simulink model "gm_parallel_8_phase_voltages"  (R2022a)
settings: Solver=FixedStepDiscrete  StartTime=0.0  StopTime=10.0  RelTol=1e-3
undefined symbols (not defined in the file or in its folder): f_c, u_dc
libraries: hdlmdlgenlib x14, simulink x2
(part 1 of 4)
settings Model: Creator=Andre Merx  LastModifiedBy=Andre Merx
settings SolverCC: AlgebraicLoopSolver=TrustRegion
settings DataIOCC: LimitDataPoints=on  SaveOutput=off  SaveTime=off
settings OptimizationCC: BlockReduction=off  ConditionallyExecuteInputs=off  DefaultParameterBehavior=Inlined  LifeSpan=inf
settings DebuggingCC: AlgebraicLoopMsg=error  InheritedTsInSrcMsg=none  SingleTaskRateTransMsg=error  UnconnectedInputMsg=warning  UnconnectedOutputMsg=warning  UnconnectedLineMsg=warning  AllowSymbolicDim=off  StrictBusMsg=ErrorOnBusTreatedAsVector  SFUnexpectedBacktrackingDiag=warning  SFNoUnconditionalDefaultTransitionDiag=warning  SFExecutionAtInitializationDiag=none  SFMachineParentedDataDiag=warning  ArithmeticOperatorsInVariantConditions=warning
settings HardwareCC: ProdBitPerPointer=32  ProdBitPerSizeT=32  ProdBitPerPtrDiffT=32  ProdLargestAtomicFloat=None  ProdIntDivRoundTo=Undefined  ProdEndianess=Unspecified  ProdWordSize=32  ProdHWDeviceType=ASIC/FPGA->ASIC/FPGA  ProdEqTarget=off
settings SFSimCC: SimUseLocalCustomCode=off  CustomCodeUndefinedFunction=UseInterfaceOnly
settings RTWCC: RTWUseLocalCustomCode=off
settings CodeAppCC: StateflowObjectComments=on
settings GRTTargetCC: TargetLangStandard=C89/C90 (ANSI)
settings ConfigComp: CovScope=ReferencedModels  CovMetricSettings=dw  CovSaveCumulativeToWorkspaceVar=on  CovSaveSingleToWorkspaceVar=on  CovExternalEMLEnable=off  CovSFcnEnable=off

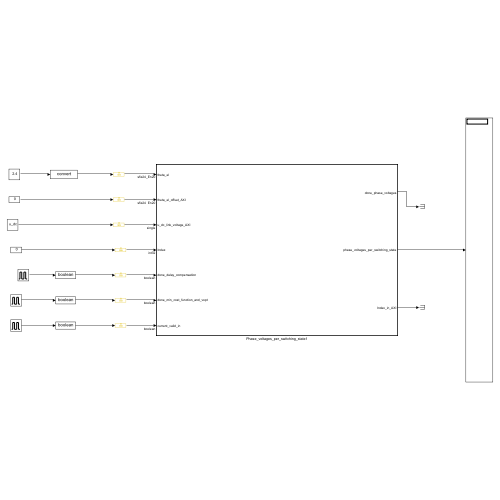
[thumbnail: Simulink's stored preview of the top-level diagram]
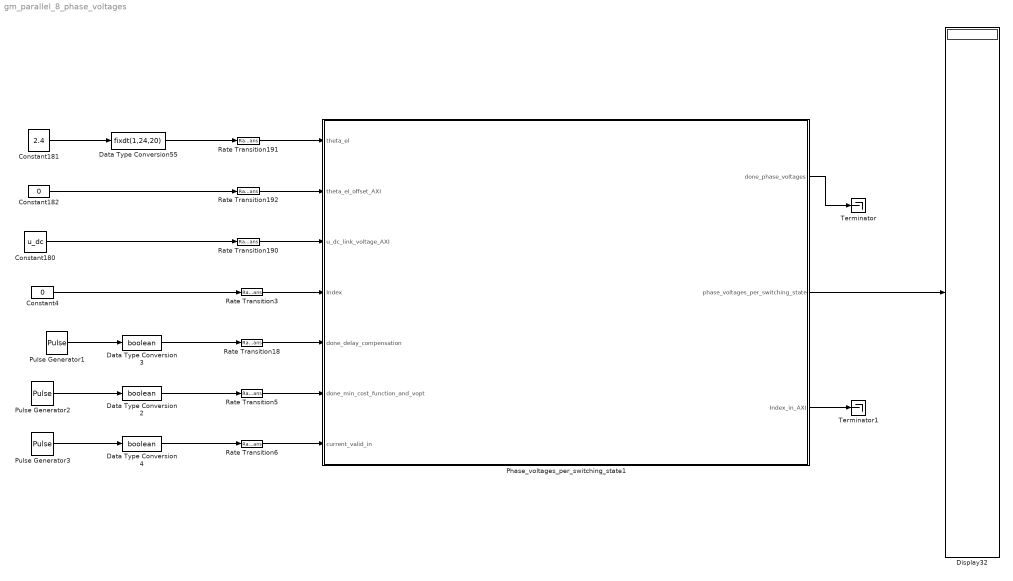
== system gm_parallel_8_phase_voltages ==
  Constant180 : Constant  Value=u_dc  OutDataTypeStr=single  SampleTime=-1
  Constant181 : Constant  Value=2.4
  Constant182 : Constant  Value=0  OutDataTypeStr=fixdt(1,24,20)  SampleTime=-1
  Constant4 : Constant  Value=0  OutDataTypeStr=int32  SampleTime=-1
  Data Type Conversion2 : DataTypeConversion  OutDataTypeStr=boolean  SaturateOnIntegerOverflow=off  RndMeth=Floor
  Data Type Conversion3 : DataTypeConversion  OutDataTypeStr=boolean  SaturateOnIntegerOverflow=off  RndMeth=Floor
  Data Type Conversion4 : DataTypeConversion  OutDataTypeStr=boolean  SaturateOnIntegerOverflow=off  RndMeth=Floor
  Data Type Conversion55 : DataTypeConversion  OutDataTypeStr=fixdt(1,24,20)  SaturateOnIntegerOverflow=off  RndMeth=Floor
  Display32 : Display
  Phase_voltages_per_switching_state1 : Subsystem  TreatAsAtomicUnit=on
  Pulse Generator1 : DiscretePulseGenerator  PulseType=Time based  Period=1/f_c
  Pulse Generator2 : DiscretePulseGenerator  PulseType=Time based  Period=1/f_c
  Pulse Generator3 : DiscretePulseGenerator  PulseType=Time based  Period=1/f_c
  Rate Transition{3,5..6,18,190..192} (7 alike) : RateTransition  OutPortSampleTime=Rt
  Terminator : Terminator
  Terminator1 : Terminator
  wires:
  Phase_voltages_per_switching_state1/3(Index_in_AXI) -> Terminator1/1
  Rate Transition3/1 -> Phase_voltages_per_switching_state1/4(Index)
  Data Type Conversion2/1 -> Rate Transition5/1
  Rate Transition6/1 -> Phase_voltages_per_switching_state1/7(current_valid_in)
  Rate Transition18/1 -> Phase_voltages_per_switching_state1/5(done_delay_compensation)
  Data Type Conversion3/1 -> Rate Transition18/1
  Data Type Conversion4/1 -> Rate Transition6/1
  Constant4/1 -> Rate Transition3/1
  Pulse Generator3/1 -> Data Type Conversion4/1
  Pulse Generator1/1 -> Data Type Conversion3/1
  Rate Transition5/1 -> Phase_voltages_per_switching_state1/6(done_min_cost_function_and_vopt)
  Pulse Generator2/1 -> Data Type Conversion2/1
  Phase_voltages_per_switching_state1/1(done_phase_voltages) -> Terminator/1
  Rate Transition190/1 -> Phase_voltages_per_switching_state1/3(u_dc_link_voltage_AXI)
  Rate Transition191/1 -> Phase_voltages_per_switching_state1/1(theta_el)
  Phase_voltages_per_switching_state1/2(phase_voltages_per_switching_state) -> Display32/1
  Rate Transition192/1 -> Phase_voltages_per_switching_state1/2(theta_el_offset_AXI)
  Constant182/1 -> Rate Transition192/1
  Constant180/1 -> Rate Transition190/1
  Data Type Conversion55/1 -> Rate Transition191/1
  Constant181/1 -> Data Type Conversion55/1

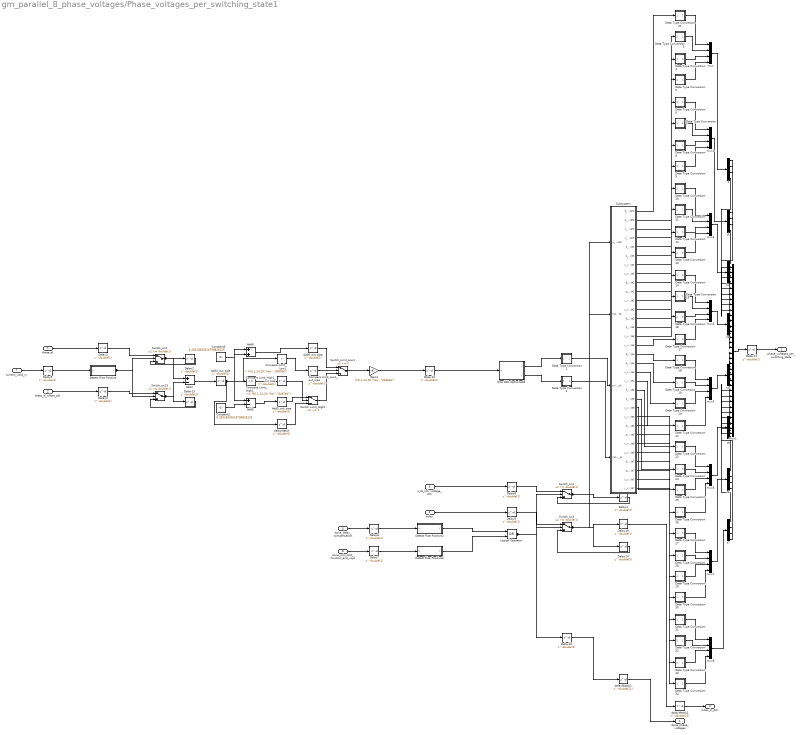
== system gm_parallel_8_phase_voltages/Phase_voltages_per_switching_state1 ==
  theta_el : Inport  OutDataTypeStr=fixdt(1, 24, 20)  PortDimensions=1  SampleTime=1e-08
  theta_el_offset_AXI : Inport  Port=2  OutDataTypeStr=fixdt(1, 24, 20)  PortDimensions=1  SampleTime=1e-08
  u_dc_link_voltage_AXI : Inport  Port=3  OutDataTypeStr=single  PortDimensions=1  SampleTime=1e-08
  Index : Inport  Port=4  OutDataTypeStr=int32  PortDimensions=1  SampleTime=1e-08
  done_delay_compensation : Inport  Port=5  OutDataTypeStr=boolean  PortDimensions=1  SampleTime=1e-08
  done_min_cost_function_and_vopt : Inport  Port=6  OutDataTypeStr=boolean  PortDimensions=1  SampleTime=1e-08
  current_valid_in : Inport  Port=7  OutDataTypeStr=boolean  PortDimensions=1  SampleTime=1e-08
  Add4 : Sum  Inputs=+-  AccumDataTypeStr=fixdt(1, 24, 20)  OutDataTypeStr=fixdt(1, 24, 20)  SampleTime=1e-08
  Add4_out_pipe : Delay  DelayLength=double(1)  InitialCondition=0  SampleTime=1e-08
  Add5 : Sum  Inputs=+-  AccumDataTypeStr=fixdt(1, 24, 20)  OutDataTypeStr=fixdt(1, 24, 20)  SampleTime=1e-08
  Add5_out_pipe : Delay  DelayLength=double(1)  InitialCondition=0  SampleTime=1e-08
  Add6 : Sum  AccumDataTypeStr=fixdt(1, 24, 20)  OutDataTypeStr=fixdt(1, 24, 20)  SampleTime=1e-08
  Add6_out_pipe : Delay  DelayLength=double(1)  InitialCondition=0  SampleTime=1e-08
  Compare Limit_High1 : simulink/Logic and Bit Operations/Compare To Constant  relop=>=  const="fi(0,1,24,20,\"hex\",\"6487ed\")"  OutDataTypeStr=boolean
  Compare Limit_High1_out_pipe : Delay  DelayLength=double(1)  InitialCondition=0  SampleTime=1e-08
  Compare Limit_Low1 : simulink/Logic and Bit Operations/Compare To Constant  relop=<  const="fi(0,1,24,20,\"hex\",\"000000\")"  OutDataTypeStr=boolean
  Compare Limit_Low1_out_pipe : Delay  DelayLength=double(1)  InitialCondition=0  SampleTime=1e-08
  Constant2 : Constant  Value=6.28318500518798828125  OutDataTypeStr=fixdt(1, 24, 20)  SampleTime=1e-08
  Constant3 : Constant  Value=6.28318500518798828125  OutDataTypeStr=fixdt(1, 24, 20)  SampleTime=1e-08
  Data Type Conversion1 : Subsystem
      mask Display: disp('NFP\nconv');
  Data Type Conversion10 : Subsystem
      mask Display: disp('NFP\nconv');
  Data Type Conversion11 : Subsystem
      mask Display: disp('NFP\nconv');
  Data Type Conversion12 : Subsystem
      mask Display: disp('NFP\nconv');
  Data Type Conversion13 : Subsystem
      mask Display: disp('NFP\nconv');
  Data Type Conversion14 : Subsystem
      mask Display: disp('NFP\nconv');
  Data Type Conversion15 : Subsystem
      mask Display: disp('NFP\nconv');
  Data Type Conversion16 : Subsystem
      mask Display: disp('NFP\nconv');
  Data Type Conversion17 : Subsystem
      mask Display: disp('NFP\nconv');
  Data Type Conversion18 : Subsystem
      mask Display: disp('NFP\nconv');
  Data Type Conversion19 : Subsystem
      mask Display: disp('NFP\nconv');
  Data Type Conversion2 : Subsystem
      mask Display: disp('NFP\nconv');
  Data Type Conversion20 : Subsystem
      mask Display: disp('NFP\nconv');
  Data Type Conversion21 : Subsystem
      mask Display: disp('NFP\nconv');
  Data Type Conversion22 : Subsystem
      mask Display: disp('NFP\nconv');
  Data Type Conversion23 : Subsystem
      mask Display: disp('NFP\nconv');
  Data Type Conversion24 : Subsystem
      mask Display: disp('NFP\nconv');
  Data Type Conversion25 : Subsystem
      mask Display: disp('NFP\nconv');
  Data Type Conversion26 : Subsystem
      mask Display: disp('NFP\nconv');
  Data Type Conversion27 : Subsystem
      mask Display: disp('NFP\nconv');
  Data Type Conversion28 : Subsystem
      mask Display: disp('NFP\nconv');
  Data Type Conversion29 : Subsystem
      mask Display: disp('NFP\nconv');
  Data Type Conversion3 : Subsystem
      mask Display: disp('NFP\nconv');
  Data Type Conversion30 : Subsystem
      mask Display: disp('NFP\nconv');
  Data Type Conversion31 : Subsystem
      mask Display: disp('NFP\nconv');
  Data Type Conversion32 : Subsystem
      mask Display: disp('NFP\nconv');
  Data Type Conversion33 : Subsystem
      mask Display: disp('NFP\nconv');
  Data Type Conversion34 : Subsystem
      mask Display: disp('NFP\nconv');
  Data Type Conversion4 : Subsystem
      mask Display: disp('NFP\nconv');
  Data Type Conversion5 : Subsystem
      mask Display: disp('NFP\nconv');
  Data Type Conversion6 : Subsystem
      mask Display: disp('NFP\nconv');
  Data Type Conversion7 : Subsystem
      mask Display: disp('NFP\nconv');
  Data Type Conversion8 : Subsystem
      mask Display: disp('NFP\nconv');
  Data Type Conversion9 : Subsystem
      mask Display: disp('NFP\nconv');
  Delay{1..14,49} (15 alike) : Delay  DelayLength=double(1)  InitialCondition=0  SampleTime=1e-08
  Detect Rise Positive : Subsystem  mask(Detect Rise Positive){vinit=double(0), InputProcessing=Elements as channels (sample based), OutDataTypeStr=boolean}
      mask prompts: vinit "Simulink:masks:InitialCondition_MP"; InputProcessing "Simulink:masks:InputProcessing_MP"; OutDataTypeStr "Simulink:masks:OutputDataType_MP"
      mask help: Simulink:masks:DetectRisePositive_MD
      mask init:
      | InputProcessing = 'Elements as channels (sample based)';
      | OutDataTypeStr = 'boolean';
      | vinit = double(0);
      mask TypeOptions InputProcessing: Simulink:masks:ColumnsAsChannelsFrameBased | Simulink:masks:ElementsAsChannelsSampleBased
      mask TypeOptions OutDataTypeStr: Simulink:masks:uint8 | Simulink:masks:boolean
      mask Display: fprintf('U > 0\n&  NOT\nU/z > 0')
  Detect Rise Positive2 : Subsystem  mask(Detect Rise Positive){vinit=double(0), InputProcessing=Elements as channels (sample based), OutDataTypeStr=boolean}
      mask prompts: vinit "Simulink:masks:InitialCondition_MP"; InputProcessing "Simulink:masks:InputProcessing_MP"; OutDataTypeStr "Simulink:masks:OutputDataType_MP"
      mask help: Simulink:masks:DetectRisePositive_MD
      mask init:
      | InputProcessing = 'Elements as channels (sample based)';
      | OutDataTypeStr = 'boolean';
      | vinit = double(0);
      mask TypeOptions InputProcessing: Simulink:masks:ColumnsAsChannelsFrameBased | Simulink:masks:ElementsAsChannelsSampleBased
      mask TypeOptions OutDataTypeStr: Simulink:masks:uint8 | Simulink:masks:boolean
      mask Display: fprintf('U > 0\n&  NOT\nU/z > 0')
  Detect Rise Positive3 : Subsystem  mask(Detect Rise Positive){vinit=double(0), InputProcessing=Elements as channels (sample based), OutDataTypeStr=boolean}
      mask prompts: vinit "Simulink:masks:InitialCondition_MP"; InputProcessing "Simulink:masks:InputProcessing_MP"; OutDataTypeStr "Simulink:masks:OutputDataType_MP"
      mask help: Simulink:masks:DetectRisePositive_MD
      mask init:
      | InputProcessing = 'Elements as channels (sample based)';
      | OutDataTypeStr = 'boolean';
      | vinit = double(0);
      mask TypeOptions InputProcessing: Simulink:masks:ColumnsAsChannelsFrameBased | Simulink:masks:ElementsAsChannelsSampleBased
      mask TypeOptions OutDataTypeStr: Simulink:masks:uint8 | Simulink:masks:boolean
      mask Display: fprintf('U > 0\n&  NOT\nU/z > 0')
  Gain1 : Gain  Gain="fi(0,1,24,20,\"hex\",\"028be6\")"  ParamDataTypeStr=fixdt(1, 24, 20)  OutDataTypeStr=fixdt(1, 24, 20)  SampleTime=1e-08
  Logical Operator : Logic  Operator=OR  AllPortsSameDT=off  OutDataTypeStr=boolean  SampleTime=1e-08
  Sine HDL Optimized2 : Subsystem  mask(Sine and Cosine HDL optimized block){OutputFormula=sin(2*pi*u) and cos(2*pi*u), NumDataPoints=double(512), TableDataTypeStr=fixdt(1,15,14), SimulateLUTROMDelay=off}
      mask prompts: OutputFormula "Simulink:masks:OutputFormula_MP"; NumDataPoints "HDLShared:hdlshared:CosineHDL_Npts"; TableDataTypeStr "Simulink:blkprm_prompts:TABLE_UNIFIEDDATATYPE"; SimulateLUTROMDelay "HDLShared:hdlshared:CosineHDL_SimulateLUTDelay"
      mask help: Sine and Cosine HDL optimized block using quarter wave symmetry, and HDL friendly settings.
      mask Help: helpview([docroot '/hdlcoder/helptargets.map'],'SineAndCosineHDL_Optimized');
      mask TypeOptions OutputFormula: sin(2*pi*u) | cos(2*pi*u) | exp(j*2*pi*u) | sin(2*pi*u) and cos(2*pi*u)
      mask Display:
      | port_label('input',1,'u')
      | port_label('output',1,'sin(2*pi*u)')
      | port_label('output',2,'cos(2*pi*u)')
      | xpos = 0.35;
      | yoffset = 0.5;
      | if ( SimulateLUTROMDelay )
      |   text(xpos,yoffset,'HDL (Z^{-1})','texmode','on')
      | else
      |    text(xpos,yoffset,'HDL')
      | end
  Subsystem : Subsystem
  Switch_Limit_High1 : Switch  Criteria=u2 ~= 0  Threshold=double(0)  OutDataTypeStr=fixdt(1, 24, 20)  SampleTime=1e-08  SaturateOnIntegerOverflow=off  InputSameDT=off
  Switch_Limit_Low1 : Switch  Criteria=u2 ~= 0  Threshold=double(0)  OutDataTypeStr=fixdt(1, 24, 20)  SampleTime=1e-08  SaturateOnIntegerOverflow=off  InputSameDT=off
  Switch_on1 : Switch  Threshold=double(1)  OutDataTypeStr=single  RndMeth=Simplest  SampleTime=1e-08  SaturateOnIntegerOverflow=off  InputSameDT=off
  Switch_on13 : Switch  Threshold=double(1)  OutDataTypeStr=fixdt(1, 24, 20)  RndMeth=Simplest  SampleTime=1e-08  SaturateOnIntegerOverflow=off  InputSameDT=off
  Switch_on2 : Switch  Threshold=double(1)  OutDataTypeStr=fixdt(1, 24, 20)  RndMeth=Simplest  SampleTime=1e-08  SaturateOnIntegerOverflow=off  InputSameDT=off
  Switch_on3 : Switch  Threshold=double(1)  OutDataTypeStr=int32  RndMeth=Simplest  SampleTime=1e-08  SaturateOnIntegerOverflow=off  InputSameDT=off
  delayMatch : Delay  DelayLength=double(1)  InitialCondition=0  SampleTime=1e-08
  delayMatch1 : Delay  DelayLength=double(21)  InitialCondition=0  SampleTime=1e-08
  delayMatch2 : Delay  DelayLength=double(21)  InitialCondition=0  SampleTime=1e-08
  mux{,2..8} (8 alike) : Mux
  mux1 : Mux  Inputs=32
  t{,1..7} (8 alike) : Demux
  done_phase_voltages : Outport  SampleTime=1e-08
  phase_voltages_per_switching_state : Outport  Port=2  SampleTime=1e-08
  Index_in_AXI : Outport  Port=3  SampleTime=1e-08
  wires:
  theta_el/1 -> Delay3/1
  theta_el_offset_AXI/1 -> Delay4/1
  u_dc_link_voltage_AXI/1 -> Delay8/1
  Index/1 -> Delay9/1
  done_delay_compensation/1 -> Delay6/1
  done_min_cost_function_and_vopt/1 -> Delay7/1
  current_valid_in/1 -> Delay5/1
  delayMatch/1 -> Switch_Limit_High1/3
  Add5_out_pipe/1 -> Switch_Limit_High1/1
  Add6_out_pipe/1 -> Switch_Limit_Low1/1
  Compare Limit_High1_out_pipe/1 -> Switch_Limit_High1/2
  Compare Limit_Low1_out_pipe/1 -> Switch_Limit_Low1/2
  Constant2/1 -> Add5/2
  Constant3/1 -> Add6/2
  delayMatch1/1 -> done_phase_voltages/1
  Delay11/1 -> phase_voltages_per_switching_state/1
  Delay12/1 -> Sine HDL Optimized2/1(u)
  Delay3/1 -> Switch_on2/1
  Delay4/1 -> Switch_on13/1
  delayMatch2/1 -> Index_in_AXI/1
  Delay5/1 -> Detect Rise Positive/1(U)
  Delay6/1 -> Detect Rise Positive2/1(U)
  Delay7/1 -> Detect Rise Positive3/1(U)
  Delay8/1 -> Switch_on1/1
  Delay9/1 -> Switch_on3/1
  Detect Rise Positive/1(Y) -> Switch_on2/2, Switch_on13/2
  Detect Rise Positive2/1(Y) -> Logical Operator/1
  Detect Rise Positive3/1(Y) -> Logical Operator/2
  Gain1/1 -> Delay12/1
  Logical Operator/1 -> Delay10/1, Switch_on1/2, Switch_on3/2
  mux/1 -> t/1
  mux1/1 -> Delay11/1
  mux2/1 -> t1/1
  mux3/1 -> t2/1
  mux4/1 -> t3/1
  mux5/1 -> t4/1
  mux6/1 -> t5/1
  mux7/1 -> t6/1
  mux8/1 -> t7/1
  Sine HDL Optimized2/1(x) -> Data Type Conversion1/1(In1)
  Sine HDL Optimized2/2(y) -> Data Type Conversion2/1(In1)
  Subsystem/1(d_voltage_per_switching_state) -> Data Type Conversion21/1(In1)
  Subsystem/2(q_voltage_per_switching_state) -> Data Type Conversion3/1(In1)
  Subsystem/3(x_voltage_per_switching_state) -> Data Type Conversion4/1(In1)
  Subsystem/4(y_voltage_per_switching_state) -> Data Type Conversion5/1(In1)
  Subsystem/5(d_voltage_per_switching_state1) -> Data Type Conversion6/1(In1)
  Subsystem/6(q_voltage_per_switching_state1) -> Data Type Conversion7/1(In1)
  Subsystem/7(x_voltage_per_switching_state1) -> Data Type Conversion8/1(In1)
  Subsystem/8(y_voltage_per_switching_state1) -> Data Type Conversion9/1(In1)
  Subsystem/9(d_voltage_per_switching_state2) -> Data Type Conversion10/1(In1)
  Subsystem/10(q_voltage_per_switching_state2) -> Data Type Conversion11/1(In1)
  Subsystem/11(x_voltage_per_switching_state2) -> Data Type Conversion12/1(In1)
  Subsystem/12(y_voltage_per_switching_state2) -> Data Type Conversion13/1(In1)
  Subsystem/13(d_voltage_per_switching_state3) -> Data Type Conversion14/1(In1)
  Subsystem/14(q_voltage_per_switching_state3) -> Data Type Conversion15/1(In1)
  Subsystem/15(x_voltage_per_switching_state3) -> Data Type Conversion16/1(In1)
  Subsystem/16(y_voltage_per_switching_state3) -> Data Type Conversion17/1(In1)
  Subsystem/17(d_voltage_per_switching_state4) -> Data Type Conversion18/1(In1)
  Subsystem/18(q_voltage_per_switching_state4) -> Data Type Conversion19/1(In1)
  Subsystem/19(x_voltage_per_switching_state4) -> Data Type Conversion20/1(In1)
  Subsystem/20(y_voltage_per_switching_state4) -> Data Type Conversion22/1(In1)
  Subsystem/21(d_voltage_per_switching_state5) -> Data Type Conversion23/1(In1)
  Subsystem/22(q_voltage_per_switching_state5) -> Data Type Conversion24/1(In1)
  Subsystem/23(x_voltage_per_switching_state5) -> Data Type Conversion25/1(In1)
  Subsystem/24(y_voltage_per_switching_state5) -> Data Type Conversion26/1(In1)
  Subsystem/25(d_voltage_per_switching_state6) -> Data Type Conversion27/1(In1)
  Subsystem/26(q_voltage_per_switching_state6) -> Data Type Conversion28/1(In1)
  Subsystem/27(x_voltage_per_switching_state6) -> Data Type Conversion29/1(In1)
  Subsystem/28(y_voltage_per_switching_state6) -> Data Type Conversion30/1(In1)
  Subsystem/29(d_voltage_per_switching_state7) -> Data Type Conversion31/1(In1)
  Subsystem/30(q_voltage_per_switching_state7) -> Data Type Conversion32/1(In1)
  Subsystem/31(x_voltage_per_switching_state7) -> Data Type Conversion33/1(In1)
  Subsystem/32(y_voltage_per_switching_state7) -> Data Type Conversion34/1(In1)
  Switch_Limit_High1/1 -> Switch_Limit_Low1/3
  Switch_Limit_Low1/1 -> Gain1/1
  Switch_on1/1 -> Subsystem/1(u_dc_link_voltage15), Delay1/1
  Switch_on13/1 -> Add4/2, Delay13/1
  Switch_on2/1 -> Add4/1, Delay2/1
  Switch_on3/1 -> Delay49/1, Subsystem/2(Index 15), Delay14/1
  Add4/1 -> Add4_out_pipe/1
  Add5/1 -> Add5_out_pipe/1
  Add6/1 -> Add6_out_pipe/1
  Compare Limit_High1/1 -> Compare Limit_High1_out_pipe/1
  Compare Limit_Low1/1 -> Compare Limit_Low1_out_pipe/1
  t/1 -> mux1/1
  t/2 -> mux1/2
  t/3 -> mux1/3
  t/4 -> mux1/4
  t1/1 -> mux1/5
  t1/2 -> mux1/6
  t1/3 -> mux1/7
  t1/4 -> mux1/8
  t2/1 -> mux1/9
  t2/2 -> mux1/10
  t2/3 -> mux1/11
  t2/4 -> mux1/12
  t3/1 -> mux1/13
  t3/2 -> mux1/14
  t3/3 -> mux1/15
  t3/4 -> mux1/16
  t4/1 -> mux1/17
  t4/2 -> mux1/18
  t4/3 -> mux1/19
  t4/4 -> mux1/20
  t5/1 -> mux1/21
  t5/2 -> mux1/22
  t5/3 -> mux1/23
  t5/4 -> mux1/24
  t6/1 -> mux1/25
  t6/2 -> mux1/26
  t6/3 -> mux1/27
  t6/4 -> mux1/28
  t7/1 -> mux1/29
  t7/2 -> mux1/30
  t7/3 -> mux1/31
  t7/4 -> mux1/32
  Add4_out_pipe/1 -> delayMatch/1, Compare Limit_Low1/1, Compare Limit_High1/1, Add6/1, Add5/1
  Delay10/1 -> delayMatch1/1
  Delay49/1 -> delayMatch2/1
  Data Type Conversion1/1(Out1) -> Subsystem/3(sin_theta_el)
  Data Type Conversion10/1(Out1) -> mux3/1
  Data Type Conversion11/1(Out1) -> mux3/2
  Data Type Conversion12/1(Out1) -> mux3/3
  Data Type Conversion13/1(Out1) -> mux3/4
  Data Type Conversion14/1(Out1) -> mux4/1
  Data Type Conversion15/1(Out1) -> mux4/2
  Data Type Conversion16/1(Out1) -> mux4/3
  Data Type Conversion17/1(Out1) -> mux4/4
  Data Type Conversion18/1(Out1) -> mux5/1
  Data Type Conversion19/1(Out1) -> mux5/2
  Data Type Conversion2/1(Out1) -> Subsystem/4(cos_theta_el)
  Data Type Conversion20/1(Out1) -> mux5/3
  Data Type Conversion21/1(Out1) -> mux/1
  Data Type Conversion22/1(Out1) -> mux5/4
  Data Type Conversion23/1(Out1) -> mux6/1
  Data Type Conversion24/1(Out1) -> mux6/2
  Data Type Conversion25/1(Out1) -> mux6/3
  Data Type Conversion26/1(Out1) -> mux6/4
  Data Type Conversion27/1(Out1) -> mux7/1
  Data Type Conversion28/1(Out1) -> mux7/2
  Data Type Conversion29/1(Out1) -> mux7/3
  Data Type Conversion3/1(Out1) -> mux/2
  Data Type Conversion30/1(Out1) -> mux7/4
  Data Type Conversion31/1(Out1) -> mux8/1
  Data Type Conversion32/1(Out1) -> mux8/2
  Data Type Conversion33/1(Out1) -> mux8/3
  Data Type Conversion34/1(Out1) -> mux8/4
  Data Type Conversion4/1(Out1) -> mux/3
  Data Type Conversion5/1(Out1) -> mux/4
  Data Type Conversion6/1(Out1) -> mux2/1
  Data Type Conversion7/1(Out1) -> mux2/2
  Data Type Conversion8/1(Out1) -> mux2/3
  Data Type Conversion9/1(Out1) -> mux2/4
  Delay1/1 -> Switch_on1/3
  Delay14/1 -> Switch_on3/3
  Delay2/1 -> Switch_on2/3
  Delay13/1 -> Switch_on13/3

== system gm_parallel_8_phase_voltages/Phase_voltages_per_switching_state1/Data Type Conversion1 ==
  In1 : Inport
  Data Type Conversion1 : DataTypeConversion  OutDataTypeStr=single  SampleTime=1e-08  SaturateOnIntegerOverflow=off  RndMeth=Floor
  Data Type Conversion1_pd1 : Delay  DelayLength=6
  Out1 : Outport
  wires:
  In1/1 -> Data Type Conversion1/1
  Data Type Conversion1/1 -> Data Type Conversion1_pd1/1
  Data Type Conversion1_pd1/1 -> Out1/1

== system gm_parallel_8_phase_voltages/Phase_voltages_per_switching_state1/Data Type Conversion10 ==
  In1 : Inport
  Data Type Conversion10 : DataTypeConversion  OutDataTypeStr=fixdt(1, 24, 11)  SampleTime=1e-08  SaturateOnIntegerOverflow=off  RndMeth=Floor
  Data Type Conversion10_pd1 : Delay  DelayLength=6
  Out1 : Outport
  wires:
  In1/1 -> Data Type Conversion10/1
  Data Type Conversion10/1 -> Data Type Conversion10_pd1/1
  Data Type Conversion10_pd1/1 -> Out1/1

== system gm_parallel_8_phase_voltages/Phase_voltages_per_switching_state1/Data Type Conversion11 ==
  In1 : Inport
  Data Type Conversion11 : DataTypeConversion  OutDataTypeStr=fixdt(1, 24, 11)  SampleTime=1e-08  SaturateOnIntegerOverflow=off  RndMeth=Floor
  Data Type Conversion11_pd1 : Delay  DelayLength=6
  Out1 : Outport
  wires:
  In1/1 -> Data Type Conversion11/1
  Data Type Conversion11/1 -> Data Type Conversion11_pd1/1
  Data Type Conversion11_pd1/1 -> Out1/1

== system gm_parallel_8_phase_voltages/Phase_voltages_per_switching_state1/Data Type Conversion12 ==
  In1 : Inport
  Data Type Conversion12 : DataTypeConversion  OutDataTypeStr=fixdt(1, 24, 11)  SampleTime=1e-08  SaturateOnIntegerOverflow=off  RndMeth=Floor
  Data Type Conversion12_pd1 : Delay  DelayLength=6
  Out1 : Outport
  wires:
  In1/1 -> Data Type Conversion12/1
  Data Type Conversion12/1 -> Data Type Conversion12_pd1/1
  Data Type Conversion12_pd1/1 -> Out1/1

== system gm_parallel_8_phase_voltages/Phase_voltages_per_switching_state1/Data Type Conversion13 ==
  In1 : Inport
  Data Type Conversion13 : DataTypeConversion  OutDataTypeStr=fixdt(1, 24, 11)  SampleTime=1e-08  SaturateOnIntegerOverflow=off  RndMeth=Floor
  Data Type Conversion13_pd1 : Delay  DelayLength=6
  Out1 : Outport
  wires:
  In1/1 -> Data Type Conversion13/1
  Data Type Conversion13/1 -> Data Type Conversion13_pd1/1
  Data Type Conversion13_pd1/1 -> Out1/1

== system gm_parallel_8_phase_voltages/Phase_voltages_per_switching_state1/Data Type Conversion14 ==
  In1 : Inport
  Data Type Conversion14 : DataTypeConversion  OutDataTypeStr=fixdt(1, 24, 11)  SampleTime=1e-08  SaturateOnIntegerOverflow=off  RndMeth=Floor
  Data Type Conversion14_pd1 : Delay  DelayLength=6
  Out1 : Outport
  wires:
  In1/1 -> Data Type Conversion14/1
  Data Type Conversion14/1 -> Data Type Conversion14_pd1/1
  Data Type Conversion14_pd1/1 -> Out1/1

== system gm_parallel_8_phase_voltages/Phase_voltages_per_switching_state1/Data Type Conversion15 ==
  In1 : Inport
  Data Type Conversion15 : DataTypeConversion  OutDataTypeStr=fixdt(1, 24, 11)  SampleTime=1e-08  SaturateOnIntegerOverflow=off  RndMeth=Floor
  Data Type Conversion15_pd1 : Delay  DelayLength=6
  Out1 : Outport
  wires:
  In1/1 -> Data Type Conversion15/1
  Data Type Conversion15/1 -> Data Type Conversion15_pd1/1
  Data Type Conversion15_pd1/1 -> Out1/1

== system gm_parallel_8_phase_voltages/Phase_voltages_per_switching_state1/Data Type Conversion16 ==
  In1 : Inport
  Data Type Conversion16 : DataTypeConversion  OutDataTypeStr=fixdt(1, 24, 11)  SampleTime=1e-08  SaturateOnIntegerOverflow=off  RndMeth=Floor
  Data Type Conversion16_pd1 : Delay  DelayLength=6
  Out1 : Outport
  wires:
  In1/1 -> Data Type Conversion16/1
  Data Type Conversion16/1 -> Data Type Conversion16_pd1/1
  Data Type Conversion16_pd1/1 -> Out1/1

== system gm_parallel_8_phase_voltages/Phase_voltages_per_switching_state1/Data Type Conversion17 ==
  In1 : Inport
  Data Type Conversion17 : DataTypeConversion  OutDataTypeStr=fixdt(1, 24, 11)  SampleTime=1e-08  SaturateOnIntegerOverflow=off  RndMeth=Floor
  Data Type Conversion17_pd1 : Delay  DelayLength=6
  Out1 : Outport
  wires:
  In1/1 -> Data Type Conversion17/1
  Data Type Conversion17/1 -> Data Type Conversion17_pd1/1
  Data Type Conversion17_pd1/1 -> Out1/1

== system gm_parallel_8_phase_voltages/Phase_voltages_per_switching_state1/Data Type Conversion18 ==
  In1 : Inport
  Data Type Conversion18 : DataTypeConversion  OutDataTypeStr=fixdt(1, 24, 11)  SampleTime=1e-08  SaturateOnIntegerOverflow=off  RndMeth=Floor
  Data Type Conversion18_pd1 : Delay  DelayLength=6
  Out1 : Outport
  wires:
  In1/1 -> Data Type Conversion18/1
  Data Type Conversion18/1 -> Data Type Conversion18_pd1/1
  Data Type Conversion18_pd1/1 -> Out1/1

== system gm_parallel_8_phase_voltages/Phase_voltages_per_switching_state1/Data Type Conversion19 ==
  In1 : Inport
  Data Type Conversion19 : DataTypeConversion  OutDataTypeStr=fixdt(1, 24, 11)  SampleTime=1e-08  SaturateOnIntegerOverflow=off  RndMeth=Floor
  Data Type Conversion19_pd1 : Delay  DelayLength=6
  Out1 : Outport
  wires:
  In1/1 -> Data Type Conversion19/1
  Data Type Conversion19/1 -> Data Type Conversion19_pd1/1
  Data Type Conversion19_pd1/1 -> Out1/1

== system gm_parallel_8_phase_voltages/Phase_voltages_per_switching_state1/Data Type Conversion2 ==
  In1 : Inport
  Data Type Conversion2 : DataTypeConversion  OutDataTypeStr=single  SampleTime=1e-08  SaturateOnIntegerOverflow=off  RndMeth=Floor
  Data Type Conversion2_pd1 : Delay  DelayLength=6
  Out1 : Outport
  wires:
  In1/1 -> Data Type Conversion2/1
  Data Type Conversion2/1 -> Data Type Conversion2_pd1/1
  Data Type Conversion2_pd1/1 -> Out1/1

== system gm_parallel_8_phase_voltages/Phase_voltages_per_switching_state1/Data Type Conversion20 ==
  In1 : Inport
  Data Type Conversion20 : DataTypeConversion  OutDataTypeStr=fixdt(1, 24, 11)  SampleTime=1e-08  SaturateOnIntegerOverflow=off  RndMeth=Floor
  Data Type Conversion20_pd1 : Delay  DelayLength=6
  Out1 : Outport
  wires:
  In1/1 -> Data Type Conversion20/1
  Data Type Conversion20/1 -> Data Type Conversion20_pd1/1
  Data Type Conversion20_pd1/1 -> Out1/1

== system gm_parallel_8_phase_voltages/Phase_voltages_per_switching_state1/Data Type Conversion21 ==
  In1 : Inport
  Data Type Conversion21 : DataTypeConversion  OutDataTypeStr=fixdt(1, 24, 11)  SampleTime=1e-08  SaturateOnIntegerOverflow=off  RndMeth=Floor
  Data Type Conversion21_pd1 : Delay  DelayLength=6
  Out1 : Outport
  wires:
  In1/1 -> Data Type Conversion21/1
  Data Type Conversion21/1 -> Data Type Conversion21_pd1/1
  Data Type Conversion21_pd1/1 -> Out1/1

== system gm_parallel_8_phase_voltages/Phase_voltages_per_switching_state1/Data Type Conversion22 ==
  In1 : Inport
  Data Type Conversion22 : DataTypeConversion  OutDataTypeStr=fixdt(1, 24, 11)  SampleTime=1e-08  SaturateOnIntegerOverflow=off  RndMeth=Floor
  Data Type Conversion22_pd1 : Delay  DelayLength=6
  Out1 : Outport
  wires:
  In1/1 -> Data Type Conversion22/1
  Data Type Conversion22/1 -> Data Type Conversion22_pd1/1
  Data Type Conversion22_pd1/1 -> Out1/1

== system gm_parallel_8_phase_voltages/Phase_voltages_per_switching_state1/Data Type Conversion23 ==
  In1 : Inport
  Data Type Conversion23 : DataTypeConversion  OutDataTypeStr=fixdt(1, 24, 11)  SampleTime=1e-08  SaturateOnIntegerOverflow=off  RndMeth=Floor
  Data Type Conversion23_pd1 : Delay  DelayLength=6
  Out1 : Outport
  wires:
  In1/1 -> Data Type Conversion23/1
  Data Type Conversion23/1 -> Data Type Conversion23_pd1/1
  Data Type Conversion23_pd1/1 -> Out1/1

== system gm_parallel_8_phase_voltages/Phase_voltages_per_switching_state1/Data Type Conversion24 ==
  In1 : Inport
  Data Type Conversion24 : DataTypeConversion  OutDataTypeStr=fixdt(1, 24, 11)  SampleTime=1e-08  SaturateOnIntegerOverflow=off  RndMeth=Floor
  Data Type Conversion24_pd1 : Delay  DelayLength=6
  Out1 : Outport
  wires:
  In1/1 -> Data Type Conversion24/1
  Data Type Conversion24/1 -> Data Type Conversion24_pd1/1
  Data Type Conversion24_pd1/1 -> Out1/1

== system gm_parallel_8_phase_voltages/Phase_voltages_per_switching_state1/Data Type Conversion25 ==
  In1 : Inport
  Data Type Conversion25 : DataTypeConversion  OutDataTypeStr=fixdt(1, 24, 11)  SampleTime=1e-08  SaturateOnIntegerOverflow=off  RndMeth=Floor
  Data Type Conversion25_pd1 : Delay  DelayLength=6
  Out1 : Outport
  wires:
  In1/1 -> Data Type Conversion25/1
  Data Type Conversion25/1 -> Data Type Conversion25_pd1/1
  Data Type Conversion25_pd1/1 -> Out1/1

== system gm_parallel_8_phase_voltages/Phase_voltages_per_switching_state1/Data Type Conversion26 ==
  In1 : Inport
  Data Type Conversion26 : DataTypeConversion  OutDataTypeStr=fixdt(1, 24, 11)  SampleTime=1e-08  SaturateOnIntegerOverflow=off  RndMeth=Floor
  Data Type Conversion26_pd1 : Delay  DelayLength=6
  Out1 : Outport
  wires:
  In1/1 -> Data Type Conversion26/1
  Data Type Conversion26/1 -> Data Type Conversion26_pd1/1
  Data Type Conversion26_pd1/1 -> Out1/1

== system gm_parallel_8_phase_voltages/Phase_voltages_per_switching_state1/Data Type Conversion27 ==
  In1 : Inport
  Data Type Conversion27 : DataTypeConversion  OutDataTypeStr=fixdt(1, 24, 11)  SampleTime=1e-08  SaturateOnIntegerOverflow=off  RndMeth=Floor
  Data Type Conversion27_pd1 : Delay  DelayLength=6
  Out1 : Outport
  wires:
  In1/1 -> Data Type Conversion27/1
  Data Type Conversion27/1 -> Data Type Conversion27_pd1/1
  Data Type Conversion27_pd1/1 -> Out1/1

== system gm_parallel_8_phase_voltages/Phase_voltages_per_switching_state1/Data Type Conversion28 ==
  In1 : Inport
  Data Type Conversion28 : DataTypeConversion  OutDataTypeStr=fixdt(1, 24, 11)  SampleTime=1e-08  SaturateOnIntegerOverflow=off  RndMeth=Floor
  Data Type Conversion28_pd1 : Delay  DelayLength=6
  Out1 : Outport
  wires:
  In1/1 -> Data Type Conversion28/1
  Data Type Conversion28/1 -> Data Type Conversion28_pd1/1
  Data Type Conversion28_pd1/1 -> Out1/1

== system gm_parallel_8_phase_voltages/Phase_voltages_per_switching_state1/Data Type Conversion29 ==
  In1 : Inport
  Data Type Conversion29 : DataTypeConversion  OutDataTypeStr=fixdt(1, 24, 11)  SampleTime=1e-08  SaturateOnIntegerOverflow=off  RndMeth=Floor
  Data Type Conversion29_pd1 : Delay  DelayLength=6
  Out1 : Outport
  wires:
  In1/1 -> Data Type Conversion29/1
  Data Type Conversion29/1 -> Data Type Conversion29_pd1/1
  Data Type Conversion29_pd1/1 -> Out1/1

== system gm_parallel_8_phase_voltages/Phase_voltages_per_switching_state1/Data Type Conversion3 ==
  In1 : Inport
  Data Type Conversion3 : DataTypeConversion  OutDataTypeStr=fixdt(1, 24, 11)  SampleTime=1e-08  SaturateOnIntegerOverflow=off  RndMeth=Floor
  Data Type Conversion3_pd1 : Delay  DelayLength=6
  Out1 : Outport
  wires:
  In1/1 -> Data Type Conversion3/1
  Data Type Conversion3/1 -> Data Type Conversion3_pd1/1
  Data Type Conversion3_pd1/1 -> Out1/1

== system gm_parallel_8_phase_voltages/Phase_voltages_per_switching_state1/Data Type Conversion30 ==
  In1 : Inport
  Data Type Conversion30 : DataTypeConversion  OutDataTypeStr=fixdt(1, 24, 11)  SampleTime=1e-08  SaturateOnIntegerOverflow=off  RndMeth=Floor
  Data Type Conversion30_pd1 : Delay  DelayLength=6
  Out1 : Outport
  wires:
  In1/1 -> Data Type Conversion30/1
  Data Type Conversion30/1 -> Data Type Conversion30_pd1/1
  Data Type Conversion30_pd1/1 -> Out1/1

== system gm_parallel_8_phase_voltages/Phase_voltages_per_switching_state1/Data Type Conversion31 ==
  In1 : Inport
  Data Type Conversion31 : DataTypeConversion  OutDataTypeStr=fixdt(1, 24, 11)  SampleTime=1e-08  SaturateOnIntegerOverflow=off  RndMeth=Floor
  Data Type Conversion31_pd1 : Delay  DelayLength=6
  Out1 : Outport
  wires:
  In1/1 -> Data Type Conversion31/1
  Data Type Conversion31/1 -> Data Type Conversion31_pd1/1
  Data Type Conversion31_pd1/1 -> Out1/1

== system gm_parallel_8_phase_voltages/Phase_voltages_per_switching_state1/Data Type Conversion32 ==
  In1 : Inport
  Data Type Conversion32 : DataTypeConversion  OutDataTypeStr=fixdt(1, 24, 11)  SampleTime=1e-08  SaturateOnIntegerOverflow=off  RndMeth=Floor
  Data Type Conversion32_pd1 : Delay  DelayLength=6
  Out1 : Outport
  wires:
  In1/1 -> Data Type Conversion32/1
  Data Type Conversion32/1 -> Data Type Conversion32_pd1/1
  Data Type Conversion32_pd1/1 -> Out1/1

== system gm_parallel_8_phase_voltages/Phase_voltages_per_switching_state1/Data Type Conversion33 ==
  In1 : Inport
  Data Type Conversion33 : DataTypeConversion  OutDataTypeStr=fixdt(1, 24, 11)  SampleTime=1e-08  SaturateOnIntegerOverflow=off  RndMeth=Floor
  Data Type Conversion33_pd1 : Delay  DelayLength=6
  Out1 : Outport
  wires:
  In1/1 -> Data Type Conversion33/1
  Data Type Conversion33/1 -> Data Type Conversion33_pd1/1
  Data Type Conversion33_pd1/1 -> Out1/1

== system gm_parallel_8_phase_voltages/Phase_voltages_per_switching_state1/Data Type Conversion34 ==
  In1 : Inport
  Data Type Conversion34 : DataTypeConversion  OutDataTypeStr=fixdt(1, 24, 11)  SampleTime=1e-08  SaturateOnIntegerOverflow=off  RndMeth=Floor
  Data Type Conversion34_pd1 : Delay  DelayLength=6
  Out1 : Outport
  wires:
  In1/1 -> Data Type Conversion34/1
  Data Type Conversion34/1 -> Data Type Conversion34_pd1/1
  Data Type Conversion34_pd1/1 -> Out1/1

== system gm_parallel_8_phase_voltages/Phase_voltages_per_switching_state1/Data Type Conversion4 ==
  In1 : Inport
  Data Type Conversion4 : DataTypeConversion  OutDataTypeStr=fixdt(1, 24, 11)  SampleTime=1e-08  SaturateOnIntegerOverflow=off  RndMeth=Floor
  Data Type Conversion4_pd1 : Delay  DelayLength=6
  Out1 : Outport
  wires:
  In1/1 -> Data Type Conversion4/1
  Data Type Conversion4/1 -> Data Type Conversion4_pd1/1
  Data Type Conversion4_pd1/1 -> Out1/1

== system gm_parallel_8_phase_voltages/Phase_voltages_per_switching_state1/Data Type Conversion5 ==
  In1 : Inport
  Data Type Conversion5 : DataTypeConversion  OutDataTypeStr=fixdt(1, 24, 11)  SampleTime=1e-08  SaturateOnIntegerOverflow=off  RndMeth=Floor
  Data Type Conversion5_pd1 : Delay  DelayLength=6
  Out1 : Outport
  wires:
  In1/1 -> Data Type Conversion5/1
  Data Type Conversion5/1 -> Data Type Conversion5_pd1/1
  Data Type Conversion5_pd1/1 -> Out1/1

== system gm_parallel_8_phase_voltages/Phase_voltages_per_switching_state1/Data Type Conversion6 ==
  In1 : Inport
  Data Type Conversion6 : DataTypeConversion  OutDataTypeStr=fixdt(1, 24, 11)  SampleTime=1e-08  SaturateOnIntegerOverflow=off  RndMeth=Floor
  Data Type Conversion6_pd1 : Delay  DelayLength=6
  Out1 : Outport
  wires:
  In1/1 -> Data Type Conversion6/1
  Data Type Conversion6/1 -> Data Type Conversion6_pd1/1
  Data Type Conversion6_pd1/1 -> Out1/1

== system gm_parallel_8_phase_voltages/Phase_voltages_per_switching_state1/Data Type Conversion7 ==
  In1 : Inport
  Data Type Conversion7 : DataTypeConversion  OutDataTypeStr=fixdt(1, 24, 11)  SampleTime=1e-08  SaturateOnIntegerOverflow=off  RndMeth=Floor
  Data Type Conversion7_pd1 : Delay  DelayLength=6
  Out1 : Outport
  wires:
  In1/1 -> Data Type Conversion7/1
  Data Type Conversion7/1 -> Data Type Conversion7_pd1/1
  Data Type Conversion7_pd1/1 -> Out1/1

== system gm_parallel_8_phase_voltages/Phase_voltages_per_switching_state1/Data Type Conversion8 ==
  In1 : Inport
  Data Type Conversion8 : DataTypeConversion  OutDataTypeStr=fixdt(1, 24, 11)  SampleTime=1e-08  SaturateOnIntegerOverflow=off  RndMeth=Floor
  Data Type Conversion8_pd1 : Delay  DelayLength=6
  Out1 : Outport
  wires:
  In1/1 -> Data Type Conversion8/1
  Data Type Conversion8/1 -> Data Type Conversion8_pd1/1
  Data Type Conversion8_pd1/1 -> Out1/1

== system gm_parallel_8_phase_voltages/Phase_voltages_per_switching_state1/Data Type Conversion9 ==
  In1 : Inport
  Data Type Conversion9 : DataTypeConversion  OutDataTypeStr=fixdt(1, 24, 11)  SampleTime=1e-08  SaturateOnIntegerOverflow=off  RndMeth=Floor
  Data Type Conversion9_pd1 : Delay  DelayLength=6
  Out1 : Outport
  wires:
  In1/1 -> Data Type Conversion9/1
  Data Type Conversion9/1 -> Data Type Conversion9_pd1/1
  Data Type Conversion9_pd1/1 -> Out1/1

== system gm_parallel_8_phase_voltages/Phase_voltages_per_switching_state1/Detect Rise Positive ==
  note: Edge
  note: U(k)
  U : Inport  OutDataTypeStr=boolean  SampleTime=1e-08
  Delay Input1 : UnitDelay  Description=Store in Global RAM  DisableCoverage=on  InitialCondition=vinit  SampleTime=-1  HasFrameUpgradeWarning=on
  FixPt Relational Operator : RelationalOperator  Operator=>  OutDataTypeStr=boolean  ZeroCross=off  InputSameDT=off
  Positive : Subsystem  mask(Compare To Zero){relop=>, OutDataTypeStr=boolean, ZeroCross=off}
      mask prompts: relop "Simulink:masks:Operator_MP"; OutDataTypeStr "Simulink:masks:OutputDataType_MP"; ZeroCross "Simulink:masks:EnableZerocrossingDetection_MP"
      mask help: Simulink:masks:CompareToZero_MD
      mask init:
      | OutDataTypeStr = 'boolean';
      | ZeroCross = 'off';
      | blkName = 'parallel_8_phase_voltages/Phase_voltages_per_switching_state1/Detect Rise\nPositive/Positive';
      | relop = '>';
      | setValue = 'boolean';
      mask TypeOptions relop: == | ~= | < | <= | >= | >
      mask TypeOptions OutDataTypeStr: Simulink:masks:uint8 | Simulink:masks:boolean
      mask Callback ZeroCross: sl('zeroCrossEnable', gcbh);
      mask Display: disp([relop,' 0'])
  Y : Outport  SampleTime=1e-08
  wires:
  Delay Input1/1 -> FixPt Relational Operator/2
  FixPt Relational Operator/1 -> Y/1
  Positive/1(y) -> FixPt Relational Operator/1, Delay Input1/1
  U/1 -> Positive/1(u)

== system gm_parallel_8_phase_voltages/Phase_voltages_per_switching_state1/Detect Rise Positive2 ==
  note: Edge
  note: U(k)
  U : Inport  OutDataTypeStr=boolean  SampleTime=1e-08
  Delay Input1 : UnitDelay  Description=Store in Global RAM  DisableCoverage=on  InitialCondition=vinit  SampleTime=-1  HasFrameUpgradeWarning=on
  FixPt Relational Operator : RelationalOperator  Operator=>  OutDataTypeStr=boolean  ZeroCross=off  InputSameDT=off
  Positive : Subsystem  mask(Compare To Zero){relop=>, OutDataTypeStr=boolean, ZeroCross=off}
      mask prompts: relop "Simulink:masks:Operator_MP"; OutDataTypeStr "Simulink:masks:OutputDataType_MP"; ZeroCross "Simulink:masks:EnableZerocrossingDetection_MP"
      mask help: Simulink:masks:CompareToZero_MD
      mask init:
      | OutDataTypeStr = 'boolean';
      | ZeroCross = 'off';
      | blkName = 'parallel_8_phase_voltages/Phase_voltages_per_switching_state1/Detect Rise\nPositive2/Positive';
      | relop = '>';
      | setValue = 'boolean';
      mask TypeOptions relop: == | ~= | < | <= | >= | >
      mask TypeOptions OutDataTypeStr: Simulink:masks:uint8 | Simulink:masks:boolean
      mask Callback ZeroCross: sl('zeroCrossEnable', gcbh);
      mask Display: disp([relop,' 0'])
  Y : Outport  SampleTime=1e-08
  wires:
  Delay Input1/1 -> FixPt Relational Operator/2
  FixPt Relational Operator/1 -> Y/1
  Positive/1(y) -> FixPt Relational Operator/1, Delay Input1/1
  U/1 -> Positive/1(u)

== system gm_parallel_8_phase_voltages/Phase_voltages_per_switching_state1/Detect Rise Positive3 ==
  note: Edge
  note: U(k)
  U : Inport  OutDataTypeStr=boolean  SampleTime=1e-08
  Delay Input1 : UnitDelay  Description=Store in Global RAM  DisableCoverage=on  InitialCondition=vinit  SampleTime=-1  HasFrameUpgradeWarning=on
  FixPt Relational Operator : RelationalOperator  Operator=>  OutDataTypeStr=boolean  ZeroCross=off  InputSameDT=off
  Positive : Subsystem  mask(Compare To Zero){relop=>, OutDataTypeStr=boolean, ZeroCross=off}
      mask prompts: relop "Simulink:masks:Operator_MP"; OutDataTypeStr "Simulink:masks:OutputDataType_MP"; ZeroCross "Simulink:masks:EnableZerocrossingDetection_MP"
      mask help: Simulink:masks:CompareToZero_MD
      mask init:
      | OutDataTypeStr = 'boolean';
      | ZeroCross = 'off';
      | blkName = 'parallel_8_phase_voltages/Phase_voltages_per_switching_state1/Detect Rise\nPositive3/Positive';
      | relop = '>';
      | setValue = 'boolean';
      mask TypeOptions relop: == | ~= | < | <= | >= | >
      mask TypeOptions OutDataTypeStr: Simulink:masks:uint8 | Simulink:masks:boolean
      mask Callback ZeroCross: sl('zeroCrossEnable', gcbh);
      mask Display: disp([relop,' 0'])
  Y : Outport  SampleTime=1e-08
  wires:
  Delay Input1/1 -> FixPt Relational Operator/2
  FixPt Relational Operator/1 -> Y/1
  Positive/1(y) -> FixPt Relational Operator/1, Delay Input1/1
  U/1 -> Positive/1(u)
